simulink model "modeloSimulink"  (R2018b)
settings: Solver=ode4  StartTime=0.0  StopTime=100  FixedStep=0.04  RelTol=1e-3
libraries: simulink x5
settings Model: Creator=root  LastModifiedBy=root

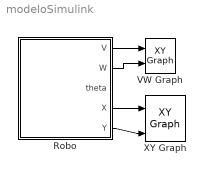
== system modeloSimulink ==
  Robo : Subsystem
  VW Graph : simulink/Sinks/XY Graph  xmin=-1  xmax=1  ymin=-2  ymax=2  st=-1
  XY Graph : simulink/Sinks/XY Graph  xmin=-1  xmax=1  ymin=-1  ymax=1  st=-1
  wires:
  Robo/1(V) -> VW Graph/1
  Robo/2(W) -> VW Graph/2
  Robo/4(X) -> XY Graph/1
  Robo/5(Y) -> XY Graph/2

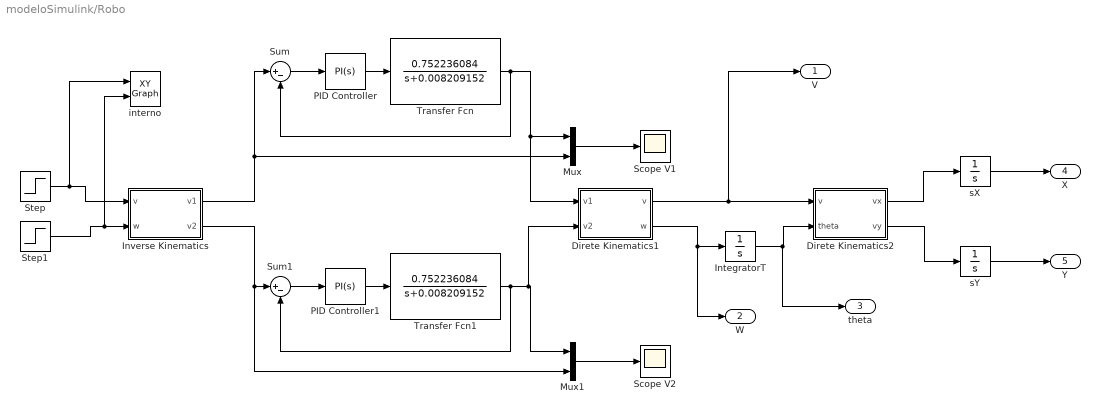
== system modeloSimulink/Robo ==
  Direte Kinematics1 : MATLAB Function  TreatAsAtomicUnit=on
  Direte Kinematics2 : MATLAB Function  TreatAsAtomicUnit=on
  IntegratorT : Integrator
  Inverse Kinematics : MATLAB Function  TreatAsAtomicUnit=on
  Mux : Mux  Inputs=2
  Mux1 : Mux  Inputs=2
  PID Controller : simulink/Continuous/PID Controller  Controller=PI  Form=Parallel  TimeDomain=Continuous-time  SampleTime=-1  IntegratorMethod=Forward Euler  FilterMethod=Forward Euler  ControllerParametersSource=internal  P=13.68  I=0.87  D=0  UseFilter=on  N=100  TunerSelectOption=Transfer Function Based (PID Tuner App)  InitialConditionSource=internal  InitialConditionForIntegrator=0  InitialConditionForFilter=0  DifferentiatorICPrevScaledInput=0  ExternalReset=none  TrackingMode=off  Kt=1  LimitOutput=off  UpperSaturationLimit=inf  LowerSaturationLimit=-inf  LinearizeAsGain=on  AntiWindupMode=none  Kb=1  POutMin=[]  POutMax=[]  IOutMin=[]  IOutMax=[]  DOutMin=[]  DOutMax=[]  NOutMin=[]  NOutMax=[]  SumOutMin=[]  SumOutMax=[]  SaturationOutMin=[]  SaturationOutMax=[]  PParamMin=[]  PParamMax=[]  IParamMin=[]  IParamMax=[]  DParamMin=[]  DParamMax=[]  NParamMin=[]  NParamMax=[]  KbParamMin=[]  KbParamMax=[]  KtParamMin=[]  KtParamMax=[]  KbOutMin=[]  KbOutMax=[]  KtOutMin=[]  KtOutMax=[]  IntegratorOutMin=[]  IntegratorOutMax=[]  FilterOutMin=[]  FilterOutMax=[]  SumI1OutMin=[]  SumI1OutMax=[]  SumI2OutMin=[]  SumI2OutMax=[]  SumI3OutMin=[]  SumI3OutMax=[]  SumI4OutMin=[]  SumI4OutMax=[]  SumDOutMin=[]  SumDOutMax=[]  DifferentiatorOutMin=[]  DifferentiatorOutMax=[]  FilterDiffOutCoefMin=[]  FilterDiffOutCoefMax=[]  ReciprocalOutMin=[]  ReciprocalOutMax=[]  SumDenOutMin=[]  SumDenOutMax=[]  SumNumOutMin=[]  SumNumOutMax=[]  DivideOutMin=[]  DivideOutMax=[]  IntegratorContinuousStateAttributes=''  IntegratorStateMustResolveToSignalObject=off  IntegratorRTWStateStorageClass=Auto  FilterContinuousStateAttributes=''  FilterStateMustResolveToSignalObject=off  FilterRTWStateStorageClass=Auto  ParallelPVariant=InternalParameters  IdealPVariant=Disabled  IVariant=InternalParameters  DVariant=Disabled  IntegratorVariant=Continuous  SatVariant=Disabled  AWVariant=Passthrough  PCopyVariant=Disabled  TRVariant=Disabled  FdbkBlocksVariant=Forward  IdealPFdbkVariant=Disabled  SatFdbkVariant=Disabled  DerivativeFilterVariant=Disabled  NVariant=Disabled  NCopyVariant=Disabled_SignalSpec  FilterICVariant=Disabled  IntegratorICVariant=InternalICs  ExternalResetVariant=Disabled  TRSumVariant=Passthrough  SumFdbkVariant=Disabled  SumVariant=Sum_PI
  PID Controller1 : simulink/Continuous/PID Controller  Controller=PI  Form=Parallel  TimeDomain=Continuous-time  SampleTime=-1  IntegratorMethod=Forward Euler  FilterMethod=Forward Euler  ControllerParametersSource=internal  P=13.68  I=0.87  D=0  UseFilter=on  N=100  TunerSelectOption=Transfer Function Based (PID Tuner App)  InitialConditionSource=internal  InitialConditionForIntegrator=0  InitialConditionForFilter=0  DifferentiatorICPrevScaledInput=0  ExternalReset=none  TrackingMode=off  Kt=1  LimitOutput=off  UpperSaturationLimit=inf  LowerSaturationLimit=-inf  LinearizeAsGain=on  AntiWindupMode=none  Kb=1  POutMin=[]  POutMax=[]  IOutMin=[]  IOutMax=[]  DOutMin=[]  DOutMax=[]  NOutMin=[]  NOutMax=[]  SumOutMin=[]  SumOutMax=[]  SaturationOutMin=[]  SaturationOutMax=[]  PParamMin=[]  PParamMax=[]  IParamMin=[]  IParamMax=[]  DParamMin=[]  DParamMax=[]  NParamMin=[]  NParamMax=[]  KbParamMin=[]  KbParamMax=[]  KtParamMin=[]  KtParamMax=[]  KbOutMin=[]  KbOutMax=[]  KtOutMin=[]  KtOutMax=[]  IntegratorOutMin=[]  IntegratorOutMax=[]  FilterOutMin=[]  FilterOutMax=[]  SumI1OutMin=[]  SumI1OutMax=[]  SumI2OutMin=[]  SumI2OutMax=[]  SumI3OutMin=[]  SumI3OutMax=[]  SumI4OutMin=[]  SumI4OutMax=[]  SumDOutMin=[]  SumDOutMax=[]  DifferentiatorOutMin=[]  DifferentiatorOutMax=[]  FilterDiffOutCoefMin=[]  FilterDiffOutCoefMax=[]  ReciprocalOutMin=[]  ReciprocalOutMax=[]  SumDenOutMin=[]  SumDenOutMax=[]  SumNumOutMin=[]  SumNumOutMax=[]  DivideOutMin=[]  DivideOutMax=[]  IntegratorContinuousStateAttributes=''  IntegratorStateMustResolveToSignalObject=off  IntegratorRTWStateStorageClass=Auto  FilterContinuousStateAttributes=''  FilterStateMustResolveToSignalObject=off  FilterRTWStateStorageClass=Auto  ParallelPVariant=InternalParameters  IdealPVariant=Disabled  IVariant=InternalParameters  DVariant=Disabled  IntegratorVariant=Continuous  SatVariant=Disabled  AWVariant=Passthrough  PCopyVariant=Disabled  TRVariant=Disabled  FdbkBlocksVariant=Forward  IdealPFdbkVariant=Disabled  SatFdbkVariant=Disabled  DerivativeFilterVariant=Disabled  NVariant=Disabled  NCopyVariant=Disabled_SignalSpec  FilterICVariant=Disabled  IntegratorICVariant=InternalICs  ExternalResetVariant=Disabled  TRSumVariant=Passthrough  SumFdbkVariant=Disabled  SumVariant=Sum_PI
  Scope V1 : Scope
  Scope V2 : Scope
  Step : Step  SampleTime=0
  Step1 : Step  After=90  SampleTime=0
  Sum : Sum  Inputs=|+-
  Sum1 : Sum  Inputs=|+-
  Transfer Fcn : TransferFcn  Numerator=[0.752236084]  Denominator=[1 0.008209152]
  Transfer Fcn1 : TransferFcn  Numerator=[0.752236084]  Denominator=[1 0.008209152]
  interno : simulink/Sinks/XY Graph  xmin=-1  xmax=1  ymin=-1  ymax=1  st=-1
  sX : Integrator
  sY : Integrator
  V : Outport
  W : Outport  Port=2
  theta : Outport  Port=3
  X : Outport  Port=4
  Y : Outport  Port=5
  wires:
  Sum/1 -> PID Controller/1
  PID Controller/1 -> Transfer Fcn/1
  Transfer Fcn/1 -> Direte Kinematics1/1(v1), Mux/1, Sum/2
  Inverse Kinematics/1(v1) -> Sum/1, Mux/2
  Mux/1 -> Scope V1/1
  Mux1/1 -> Scope V2/1
  PID Controller1/1 -> Transfer Fcn1/1
  Sum1/1 -> PID Controller1/1
  Transfer Fcn1/1 -> Direte Kinematics1/2(v2), Mux1/1, Sum1/2
  Inverse Kinematics/2(v2) -> Mux1/2, Sum1/1
  Direte Kinematics1/1(v) -> Direte Kinematics2/1(v), V/1
  Direte Kinematics1/2(w) -> W/1, IntegratorT/1
  IntegratorT/1 -> theta/1, Direte Kinematics2/2(theta)
  Direte Kinematics2/2(vy) -> sY/1
  Direte Kinematics2/1(vx) -> sX/1
  sX/1 -> X/1
  sY/1 -> Y/1
  Step/1 -> interno/1, Inverse Kinematics/1(v)
  Step1/1 -> interno/2, Inverse Kinematics/2(w)

== matlab function modeloSimulink/Robo/Direte Kinematics1 ==
  data: v1 input; v output; v2 input; w output
%function y = fcn(u)
function [v,w] = fcn(v1,v2)
    L = 2 * 0.17;
    v = (v1 + v2)/2;
    w = (v1 - v2)/L;
end

== matlab function modeloSimulink/Robo/Inverse Kinematics ==
  data: v input; v1 output; w input; v2 output
%function y = fcn(u)
function [v1,v2] = fcn(v,w)
    L = 2 * 0.17;
    v1 = v - w * L/2;
    v2 = v + w * L/2;
end

== matlab function modeloSimulink/Robo/Direte Kinematics2 ==
  data: v input; vx output; theta input; vy output
%function y = fcn(u)
function [vx,vy] = fcn(v,theta)
    vx = v * cos(deg2rad(theta));
    vy = v * sin(deg2rad(theta));
end
